simulink model "DaoBaoTin_20151230_Cau2abc"  (R2018a)
settings: Solver=FixedStepAuto  StartTime=0  StopTime=100  FixedStep=0.01  RelTol=1e-3
values from neighbouring files (symbols this model uses):
  J = 0.02    [thongso_cau2.m]
  KB = 0.015    [thongso_cau2.m]
  KF = 0.2    [thongso_cau2.m]
  KM = 0.015    [thongso_cau2.m]
  L = 0.5    [thongso_cau2.m]
  R = 2    [thongso_cau2.m]
settings Model: Creator=20151  LastModifiedBy=20151
settings DataIOCC: ReturnWorkspaceOutputs=on
settings DebuggingCC: UnconnectedInputMsg=none  UnconnectedOutputMsg=none  UnconnectedLineMsg=none  SFMachineParentedDataDiag=error
settings SFSimCC: SimUseLocalCustomCode=on
settings RTWCC: RTWUseLocalCustomCode=on

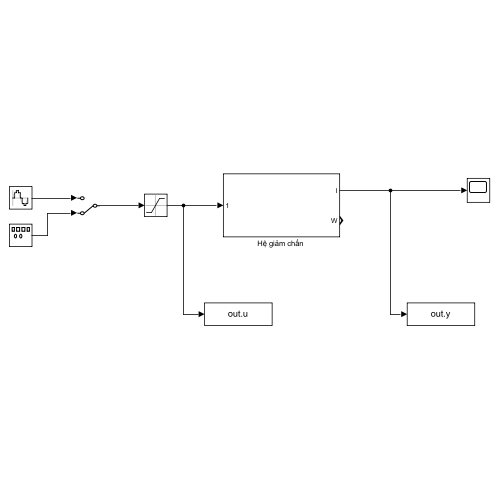
[thumbnail: Simulink's stored preview of the top-level diagram]
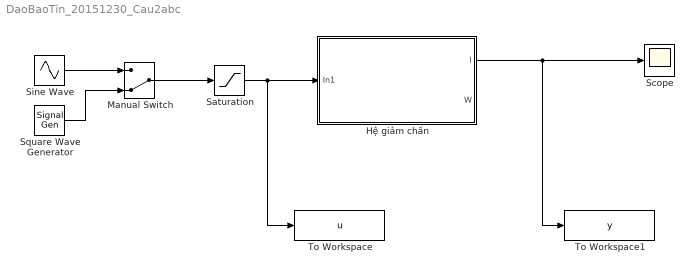
== system DaoBaoTin_20151230_Cau2abc ==
  "Hệ giảm chấn " : Subsystem
  Manual Switch : ManualSwitch  CurrentSetting=0
  Saturation : Saturate  UpperLimit=12  LowerLimit=-12
  Scope : Scope
  Sine Wave : Sin  SampleTime=0.01
  Square Wave Generator : SignalGenerator  WaveForm=random  Amplitude=20  Frequency=10  Units=rad/sec
  To Workspace : ToWorkspace  VariableName=u  SaveFormat=Timeseries  SampleTime=0.01
  To Workspace1 : ToWorkspace  VariableName=y  SaveFormat=Timeseries  SampleTime=0.01
  wires:
  Saturation/1 -> To Workspace/1, "Hệ giảm chấn "/1(In1)
  "Hệ giảm chấn "/1(I) -> To Workspace1/1, Scope/1
  Square Wave Generator/1 -> Manual Switch/2
  Manual Switch/1 -> Saturation/1
  Sine Wave/1 -> Manual Switch/1

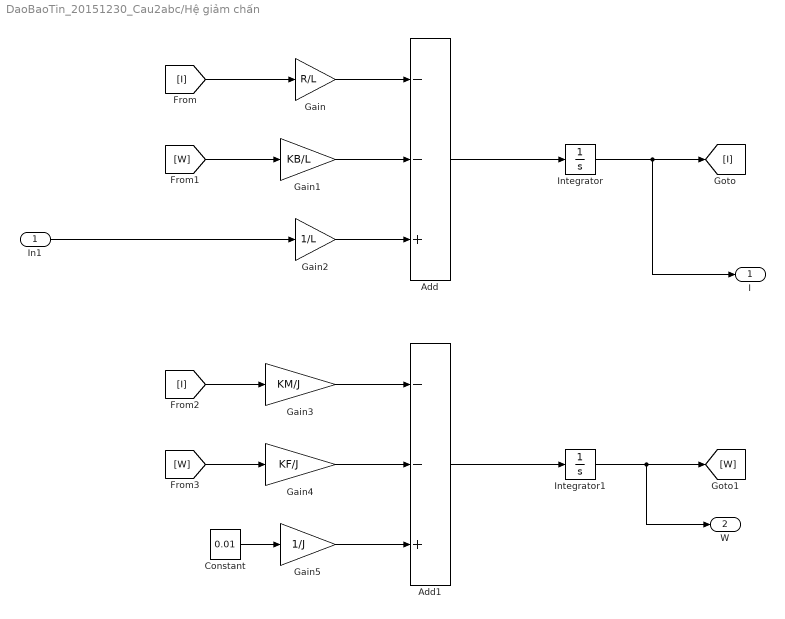
== system DaoBaoTin_20151230_Cau2abc/Hệ giảm chấn  ==
  In1 : Inport
  Add : Sum  Inputs=--+
  Add1 : Sum  Inputs=--+
  Constant : Constant  Value=0.01
  Gain : Gain  Gain=R/L
  Gain1 : Gain  Gain=KB/L
  Gain2 : Gain  Gain=1/L
  Gain3 : Gain  Gain=KM/J
  Gain4 : Gain  Gain=KF/J
  Gain5 : Gain  Gain=1/J
  Integrator : Integrator
  Integrator1 : Integrator
  I : Outport
  W : Outport  Port=2
  wires:
  Gain/1 -> Add/1
  Gain1/1 -> Add/2
  Gain2/1 -> Add/3
  Gain3/1 -> Add1/1
  Gain4/1 -> Add1/2
  Gain5/1 -> Add1/3
  Add/1 -> Integrator/1
  Add1/1 -> Integrator1/1
  Integrator/1 -> I/1, [I]
  Integrator1/1 -> W/1, [W]
  [I] -> Gain/1
  [W] -> Gain1/1
  [W] -> Gain4/1
  [I] -> Gain3/1
  In1/1 -> Gain2/1
  Constant/1 -> Gain5/1
